simulink model "SLX20231127"  (R2022b)
settings: Solver=ode4  StartTime=0.0  StopTime=20  FixedStep=.0001  RelTol=1e-3
libraries: cstblocks x2
settings Model: Creator=aghersin  LastModifiedBy=aghersin

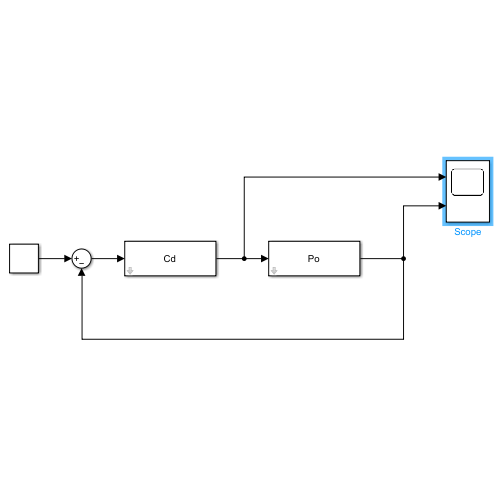
[thumbnail: Simulink's stored preview of the top-level diagram]
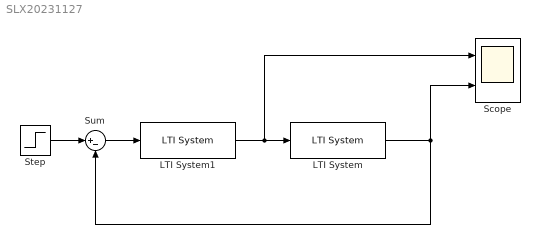
== system SLX20231127 ==
  LTI System : cstblocks/LTI System  sys=Po  IC=[]
  LTI System1 : cstblocks/LTI System  sys=Cd  IC=[]
  Scope : Scope  NumInputPorts=2
  Step : Step  SampleTime=0
  Sum : Sum  Inputs=|+-
  wires:
  LTI System1/1 -> Scope/1, LTI System/1
  Sum/1 -> LTI System1/1
  Step/1 -> Sum/1
  LTI System/1 -> Sum/2, Scope/2
